simulink model "WPT"  (Simulink 8.9)
settings: Solver=FixedStepAuto  StartTime=0.0  StopTime=1  FixedStep=1e-6  MaxStep=1e-4  RelTol=1e-3
libraries: powerlib x22
settings Model: Creator=Annai  LastModifiedBy=Annai
settings DataIOCC: LimitDataPoints=off  SaveFormat=Dataset  SignalLoggingSaveFormat=Dataset
settings OptimizationCC: LifeSpan=auto
settings DebuggingCC: UnderspecifiedInitializationDetection=Simplified  MergeDetectMultiDrivingBlocksExec=error  FcnCallInpInsideContextMsg=error  StateNameClashWarn=none  SFUnexpectedBacktrackingDiag=error  SFNoUnconditionalDefaultTransitionDiag=error  SFExecutionAtInitializationDiag=warning
settings HardwareCC: ProdBitPerPointer=64  ProdBitPerSizeT=64  ProdBitPerPtrDiffT=64  ProdLargestAtomicFloat=Float  ProdIntDivRoundTo=Zero  ProdEndianess=LittleEndian  ProdWordSize=64  ProdHWDeviceType=Intel->x86-64 (Windows64)
settings ModelReferenceCC: PropagateSignalLabelsOutOfModel=on
settings GRTTargetCC: TargetLangStandard=C99 (ISO)  GeneratePreprocessorConditionals=Use local settings  CombineOutputUpdateFcns=on  GRTInterface=off
settings ConfigComp: CovMetricSettings=dwe  CovHtmlReporting=off  CovSaveCumulativeToWorkspaceVar=off  CovSaveSingleToWorkspaceVar=off  CovExternalEMLEnable=on

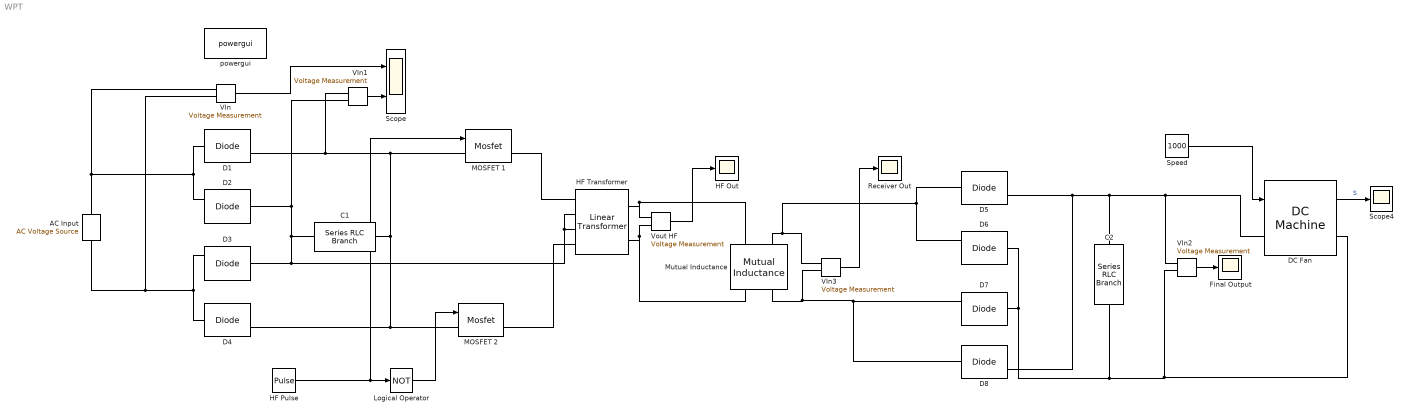
== system WPT ==
  AC Input : powerlib/Electrical Sources/AC Voltage Source  Amplitude=230  Phase=0  Frequency=50  SampleTime=0  Measurements=None  BusType=swing  Pref=10e3  Qref=0  Qmin=-inf  Qmax=+inf
  C1 : powerlib/Elements/Series RLC Branch  LConnTagsString=__new0  RConnTagsString=__new0  BranchType=C  Resistance=1  Inductance=1e-3  SetiL0=off  InitialCurrent=0  Capacitance=4700e-6  Setx0=off  InitialVoltage=0  Measurements=None
  C2 : powerlib/Elements/Series RLC Branch  LConnTagsString=__new0  RConnTagsString=__new0  BranchType=C  Resistance=1  Inductance=1e-3  SetiL0=off  InitialCurrent=0  Capacitance=1000e-6  Setx0=off  InitialVoltage=0  Measurements=None
  D{1..8} (8 alike) : powerlib/Power Electronics/Diode  Ron=0.001  Lon=0  Vf=0.8  IC=0  UseSnubber=0  Rs=500  Cs=250e-9  Measurements=on
  DC Fan : powerlib/Machines/DC Machine  PresetModel=No  MechanicalLoad=Speed w  FieldType=Permanent magnet  ShowDetailedParameters=on  MeasurementBus=off  RLa="[ 0.6  0.012]"  RLf="[ 240  120]"  Laf=1.8  MachineConstant=Torque constant (N.m/A)  Ke=1.8  Kt=.012  J=1  Bm=0  Tf=0  w0=1  Ifinit=1  TsPowergui=0  TsBlock=-1
  Final Output : Scope
  HF Out : Scope
  HF Pulse : DiscretePulseGenerator  PulseType=Time based  Period=1/25000  PulseWidth=50
  HF Transformer : powerlib/Elements/Linear Transformer  UNITS=pu  NominalPower=[ 1000 25000]  winding1="[ 15  0.002  0.08 ]"  winding2="[ 230  0.002  0.08 ]"  ThreeWindings=on  winding3=[ 230 0.002 0.08 ]  RmLm=[ 500 500 ]  Measurements=None  DataType=off
  Logical Operator : Logic  Operator=NOT  AllPortsSameDT=off  OutDataTypeStr=boolean
  MOSFET 1 : powerlib/Power Electronics/Mosfet  Ron=0.1  Lon=0  Rd=0.01  Vfd=0  IC=0  Rs=1e5  Cs=inf  Measurements=on
  MOSFET 2 : powerlib/Power Electronics/Mosfet  Ron=0.1  Lon=0  Rd=0.01  Vfd=0  IC=0  Rs=1e5  Cs=inf  Measurements=on
  Mutual Inductance : powerlib/Elements/Mutual Inductance  LConnTagsString=a|b  RConnTagsString=A|B  TypeOfMutual=Two or three windings with equal mutual terms  NumberOfWindings=2  SelfImpedance1=[1.1 1.1e-03]  SelfImpedance2=[ 1.1 1.1e-03]  ThreeWindings=off  SelfImpedance3=[ 1.1 1.1e-03]  MutualImpedance=[1.0 1.0e-03]  InductanceMatrix="[1.0 0.9  0.9 ;  0.9 1.0  0.9;  0.9 0.9 1.0 ] * 1e-3"  ResistanceMatrix="[1.0 0.9  0.9 ;  0.9 1.0  0.9;  0.9 0.9 1.0 ]"  Measurements=None
      settings: AttributesFormatString=\n  SourceProductName=Simscape Power Systems  SourceProductBaseCode=PS
  Receiver Out : Scope
  Scope : Scope  NumInputPorts=2
  Scope4 : Scope
  Speed : Constant  Value=1000
  VIn : powerlib/Measurements/Voltage Measurement  PhasorSimulation=off  OutputType=Complex  PSBequivalent=0
  VIn1 : powerlib/Measurements/Voltage Measurement  PhasorSimulation=off  OutputType=Complex  PSBequivalent=0
  VIn2 : powerlib/Measurements/Voltage Measurement  PhasorSimulation=off  OutputType=Magnitude  PSBequivalent=0
  VIn3 : powerlib/Measurements/Voltage Measurement  PhasorSimulation=off  OutputType=Magnitude  PSBequivalent=0
  Vout HF : powerlib/Measurements/Voltage Measurement  PhasorSimulation=off  OutputType=Magnitude  PSBequivalent=0
  powergui : powerlib/powergui  Priority=1  SimulationMode=Discrete  SampleTime=1e-6  frequency=60  Iterations=50  frequencyindice=0  Pbase=100e6  ErrMax=1e-4  UnitsV=kV  UnitsW=MW  buscounter=0  FunctionMessages=off  echomessages=off  EnableUseOfTLC=off  CurrentSourceSwitches=off  DisableSnubberDevices=off  DisableRonSwitches=off  DisableVfSwitches=off  DisplayEquations=off  SolverType=Tustin/Backward Euler (TBE)  Interpol=off  ExternalGateDelay=off  methode=off  Ts=100  x0status=blocks  SPID=off  SwTol=0  HookPort=off  RestoreLinks=warning  ResistiveCurrentMeasurement=off  Frange=[0:2:500]  Ylog=off  Xlog=on  ShowGrid=off  save=off  variable=ZData  structure=0  ZoomFFT=off  StartTime=0.0  cycles=1  DisplayStyle=1  fundamental=60  FreqAxis=off  MaxFrequency=1000  frequencyindicesteady=1  RmsSteady=1  display=off
  wires:
  VIn/1 -> Scope/1
  VIn1/1 -> Scope/2
  HF Pulse/1 -> Logical Operator/1, MOSFET 1/1
  Logical Operator/1 -> MOSFET 2/1
  Vout HF/1 -> HF Out/1
  VIn3/1 -> Receiver Out/1
  VIn2/1 -> Final Output/1
  Speed/1 -> DC Fan/1
  DC Fan/1 -> Scope4/1  "S"
  connections:
  D1/LConn1 -- VIn/LConn1 -- AC Input/RConn1 -- D2/RConn1
  D3/RConn1 -- AC Input/LConn1 -- VIn/LConn2 -- D4/LConn1
  D1/RConn1 -- VIn1/LConn1 -- MOSFET 1/LConn1 -- C1/LConn1 -- MOSFET 2/LConn1 -- D4/RConn1
  MOSFET 1/RConn1 -- HF Transformer/RConn4
  MOSFET 2/RConn1 -- HF Transformer/RConn1
  Vout HF/LConn1 -- Mutual Inductance/LConn1 -- HF Transformer/LConn2
  Vout HF/LConn2 -- Mutual Inductance/RConn1 -- HF Transformer/LConn1
  D2/LConn1 -- VIn1/LConn2 -- C1/RConn1 -- HF Transformer/RConn3 -- HF Transformer/RConn2 -- D3/LConn1
  VIn3/LConn1 -- Mutual Inductance/LConn2 -- D6/RConn1 -- D5/LConn1
  VIn3/LConn2 -- D7/RConn1 -- D8/LConn1 -- Mutual Inductance/RConn2
  D6/LConn1 -- DC Fan/RConn1 -- VIn2/LConn2 -- C2/RConn1 -- D7/LConn1
  D8/RConn1 -- VIn2/LConn1 -- DC Fan/LConn1 -- C2/LConn1 -- D5/RConn1
